simulink model "automated_irrigation_control_system"  (R2021a)
settings: Solver=VariableStepAuto  StartTime=0.0  StopTime=10.0  RelTol=1e-3
settings Model: Creator=YasserNet  LastModifiedBy=YasserNet

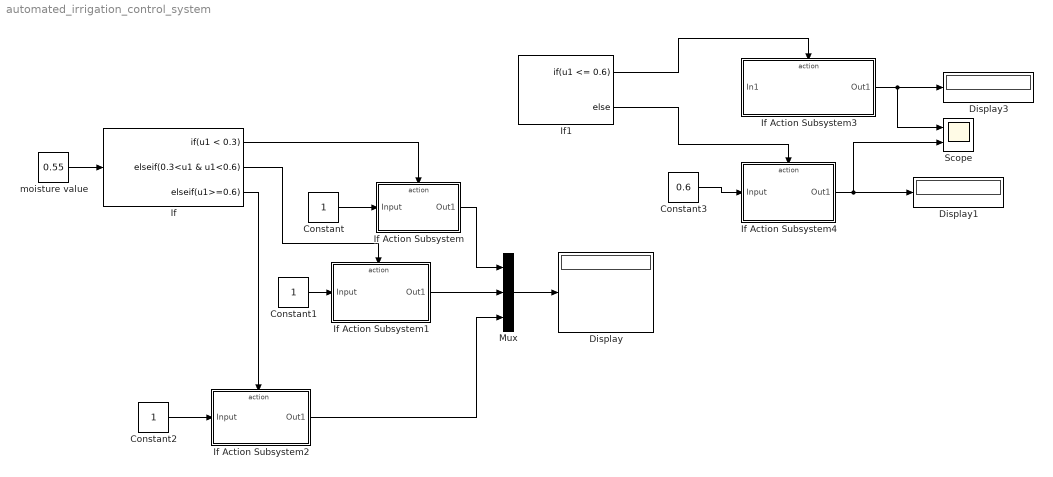
== system automated_irrigation_control_system ==
  Constant : Constant
  Constant1 : Constant
  Constant2 : Constant
  Constant3 : Constant  Value=0.6
  Display : Display
  Display1 : Display
  Display3 : Display
  If : If  IfExpression=u1 < 0.3  ElseIfExpressions="0.3<u1 & u1<0.6  ,u1>=0.6"  ShowElse=off
  If Action Subsystem : Subsystem  TreatAsAtomicUnit=on
  If Action Subsystem1 : Subsystem  TreatAsAtomicUnit=on
  If Action Subsystem2 : Subsystem  TreatAsAtomicUnit=on
  If Action Subsystem3 : Subsystem  TreatAsAtomicUnit=on
  If Action Subsystem4 : Subsystem  TreatAsAtomicUnit=on
  If1 : If  IfExpression=u1 <= 0.6
  Mux : Mux  Inputs=3
  Scope : Scope  NumInputPorts=2
  moisture value : Constant  Value=0.55
  wires:
  If/1 -> If Action Subsystem/Action
  If/2 -> If Action Subsystem1/Action
  If/3 -> If Action Subsystem2/Action
  If Action Subsystem/1(Out1) -> Mux/1
  If Action Subsystem1/1(Out1) -> Mux/2
  If Action Subsystem2/1(Out1) -> Mux/3
  Constant/1 -> If Action Subsystem/1(Input)
  Constant2/1 -> If Action Subsystem2/1(Input)
  moisture value/1 -> If/1
  If Action Subsystem3/1(Out1) -> Display3/1, Scope/1
  Constant1/1 -> If Action Subsystem1/1(Input)
  Mux/1 -> Display/1
  If1/1 -> If Action Subsystem3/Action
  If1/2 -> If Action Subsystem4/Action
  Constant3/1 -> If Action Subsystem4/1(Input)
  If Action Subsystem4/1(Out1) -> Scope/2, Display1/1

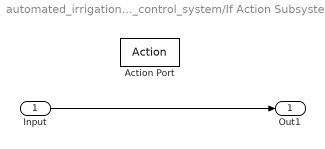
== system automated_irrigation_control_system/If Action Subsystem ==
  Input : Inport
  Action Port : ActionPort  ActionPortLabel=if(u1 < 0.3)
  Out1 : Outport
  wires:
  Input/1 -> Out1/1

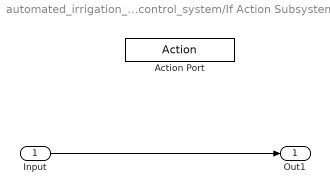
== system automated_irrigation_control_system/If Action Subsystem1 ==
  Input : Inport
  Action Port : ActionPort  ActionPortLabel="elseif(0.3<u1 & u1<0.6  )"
  Out1 : Outport
  wires:
  Input/1 -> Out1/1

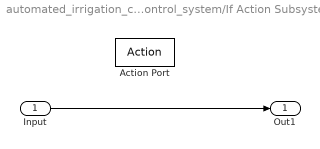
== system automated_irrigation_control_system/If Action Subsystem2 ==
  Input : Inport
  Action Port : ActionPort  ActionPortLabel=elseif(u1>=0.6)
  Out1 : Outport
  wires:
  Input/1 -> Out1/1

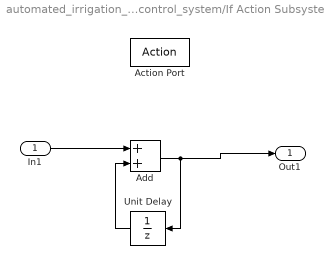
== system automated_irrigation_control_system/If Action Subsystem3 ==
  In1 : Inport
  Action Port : ActionPort  ActionPortLabel=if(u1 <= 0.6)
  Add : Sum
  Unit Delay : UnitDelay  SampleTime=-1  HasFrameUpgradeWarning=on
  Out1 : Outport
  wires:
  In1/1 -> Add/1
  Unit Delay/1 -> Add/2
  Add/1 -> Unit Delay/1, Out1/1

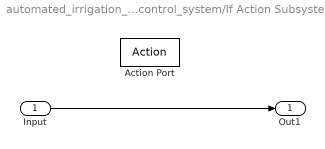
== system automated_irrigation_control_system/If Action Subsystem4 ==
  Input : Inport
  Action Port : ActionPort  ActionPortLabel=else
  Out1 : Outport
  wires:
  Input/1 -> Out1/1
